simulink model "PD_controller"  (R2016b)
settings: Solver=VariableStepAuto  StartTime=0.0  StopTime=10.0  RelTol=1e-3
values from neighbouring files (symbols this model uses):
  kd = double(subs(kdsol, [wn ksi], [0.5 0.7]))    [example1_2.m]
  kp = double(subs(kpsol, [wn ksi], [0.5 0.7]))    [example1_2.m]
undefined symbols (not defined in the file or in its folder): den, num
libraries: simulink_extras x1
settings Model: Creator=Trancemania  LastModifiedBy=Trancemania

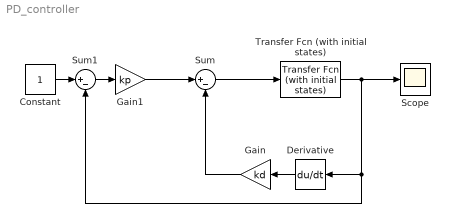
== system PD_controller ==
  Constant : Constant
  Derivative : Derivative
  Gain : Gain  Gain=kd
  Gain1 : Gain  Gain=kp
  Scope : Scope
  Sum : Sum  Inputs=|+-
  Sum1 : Sum  Inputs=|+-
  Transfer Fcn (with initial states) : simulink_extras/Additional Linear/Transfer Fcn (with initial states)  N=num  D=den  X0=0
  wires:
  Transfer Fcn (with initial states)/1 -> Scope/1, Sum1/2, Derivative/1
  Constant/1 -> Sum1/1
  Derivative/1 -> Gain/1
  Gain1/1 -> Sum/1
  Sum/1 -> Transfer Fcn (with initial states)/1
  Gain/1 -> Sum/2
  Sum1/1 -> Gain1/1
